simulink model "Admittance"  (R2023b)
settings: Solver=VariableStepAuto  StartTime=0.0  StopTime=1000  RelTol=1e-3
values from neighbouring files (symbols this model uses):
  Bm = 0.8    [Admittance_code.m]
  D = 0.6    [Admittance_code.m]
  J = 2* Jm    (= 1.836e-06)    [Admittance_code.m]
  K = 0.011    [Admittance_code.m]
  Km = K    (= 0.011)    [Admittance_code.m]
  Lw = L    (= 0.00058)    [Admittance_code.m]
  M_inv = 1/J    (= 544662.309368)    [Admittance_code.m]
  Rw = R    (= 1.17)    [Admittance_code.m]
settings Model: Creator=sayeholoumi  LastModifiedBy=sayeholoumi

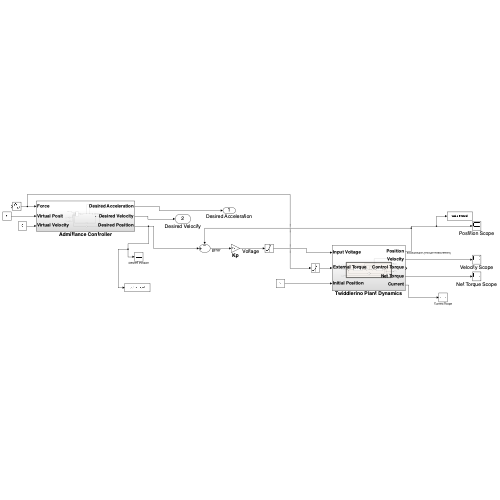
[thumbnail: Simulink's stored preview of the top-level diagram]
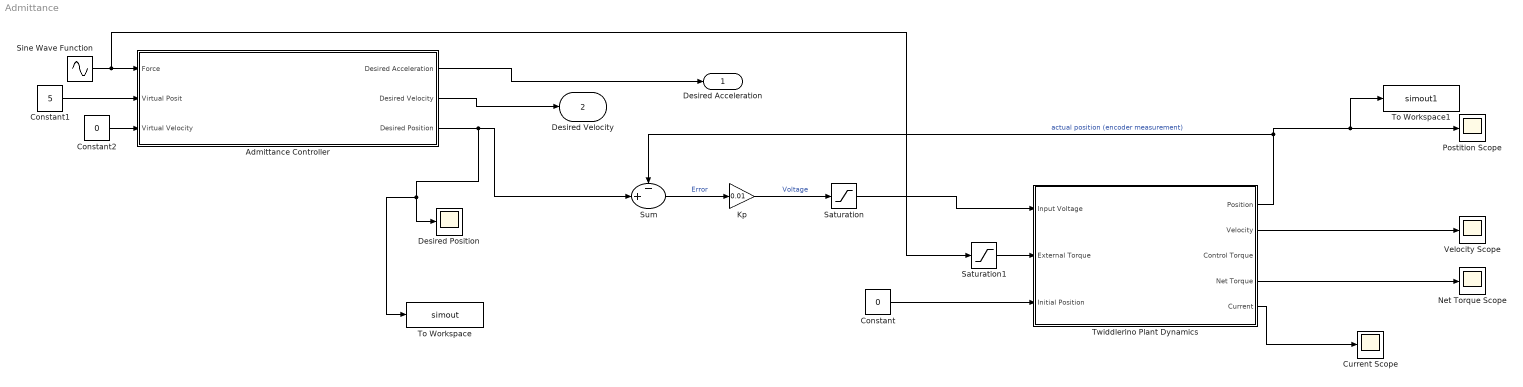
== system Admittance ==
  Admittance Controller : Subsystem
  Constant : Constant  Value=0
  Constant1 : Constant  Value=5
  Constant2 : Constant  Value=0
  Current Scope : Scope
  Desired Position : Scope
  Kp : Gain  Gain=0.01
  Net Torque Scope : Scope
  Postition Scope : Scope
  Saturation : Saturate  UpperLimit=12  LowerLimit=-12
  Saturation1 : Saturate  UpperLimit=12  LowerLimit=-12
  Sine Wave Function : Sin  TimeSource=Use external signal  SampleTime=0
  Sum : Sum  Inputs=-+|
  To Workspace : ToWorkspace  VariableName=simout  SaveFormat=Timeseries  SampleTime=-1
  To Workspace1 : ToWorkspace  VariableName=simout1  SaveFormat=Timeseries  SampleTime=-1
  Twiddlerino Plant Dynamics : Subsystem
  Velocity Scope : Scope
  Desired Acceleration : Outport
  Desired Velocity : Outport  Port=2
  wires:
  Constant/1 -> Twiddlerino Plant Dynamics/3(Initial Position)
  Twiddlerino Plant Dynamics/4(Net Torque) -> Net Torque Scope/1
  Saturation1/1 -> Twiddlerino Plant Dynamics/2(External Torque)
  Saturation/1 -> Twiddlerino Plant Dynamics/1(Input Voltage)
  Sum/1 -> Kp/1  "Error"
  Twiddlerino Plant Dynamics/1(Position) -> Sum/1, To Workspace1/1, Postition Scope/1  "actual position (encoder measurement)"
  Admittance Controller/1(Desired Acceleration) -> Desired Acceleration/1
  Sine Wave Function/1 -> Saturation1/1, Admittance Controller/1(Force)
  Twiddlerino Plant Dynamics/2(Velocity) -> Velocity Scope/1
  Admittance Controller/2(Desired Velocity) -> Desired Velocity/1
  Admittance Controller/3(Desired Position) -> To Workspace/1, Desired Position/1, Sum/2
  Twiddlerino Plant Dynamics/5(Current) -> Current Scope/1
  Kp/1 -> Saturation/1  "Voltage"
  Constant2/1 -> Admittance Controller/3(Virtual Velocity)
  Constant1/1 -> Admittance Controller/2(Virtual Posit)

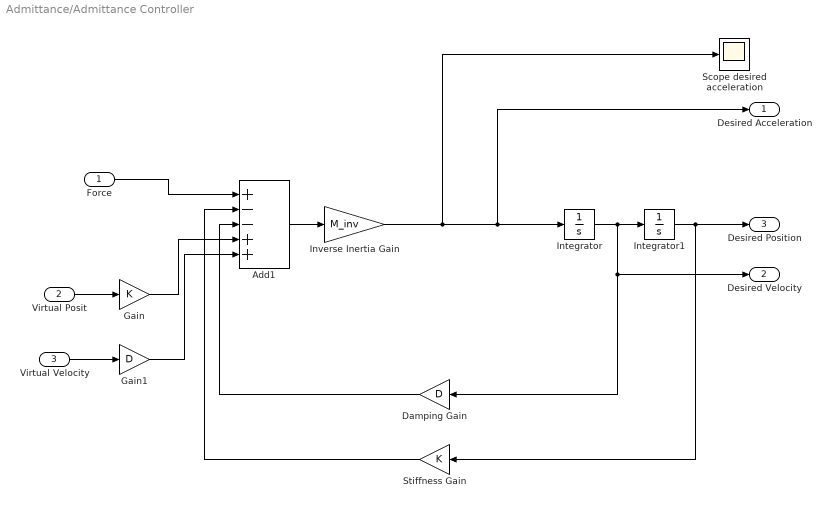
== system Admittance/Admittance Controller ==
  Force : Inport
  Virtual Posit : Inport  Port=2
  Virtual Velocity : Inport  Port=3
  Add1 : Sum  Inputs=+--++
  Damping Gain : Gain  Gain=D
  Gain : Gain  Gain=K
  Gain1 : Gain  Gain=D
  Integrator : Integrator
  Integrator1 : Integrator
  Inverse Inertia Gain : Gain  Gain=M_inv
  Scope desired acceleration : Scope
  "Stiffness Gain " : Gain  Gain=K
  Desired Acceleration : Outport
  Desired Velocity : Outport  Port=2
  Desired Position : Outport  Port=3
  wires:
  Add1/1 -> Inverse Inertia Gain/1
  Damping Gain/1 -> Add1/3
  Integrator1/1 -> Desired Position/1, "Stiffness Gain "/1
  Force/1 -> Add1/1
  Integrator/1 -> Desired Velocity/1, Damping Gain/1, Integrator1/1
  "Stiffness Gain "/1 -> Add1/2
  Inverse Inertia Gain/1 -> Scope desired acceleration/1, Desired Acceleration/1, Integrator/1
  Virtual Posit/1 -> Gain/1
  Virtual Velocity/1 -> Gain1/1
  Gain/1 -> Add1/4
  Gain1/1 -> Add1/5

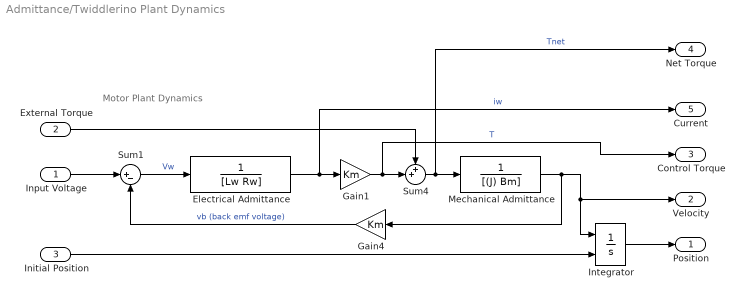
== system Admittance/Twiddlerino Plant Dynamics ==
  note: Motor Plant Dynamics
  Input Voltage : Inport
  External Torque : Inport  Port=2
  Initial Position : Inport  Port=3
  Electrical Admittance : TransferFcn  Denominator=[Lw Rw]
  Gain1 : Gain  Gain=Km
  Gain4 : Gain  Gain=Km
  Integrator : Integrator  InitialConditionSource=external
  Mechanical Admittance : TransferFcn  Denominator=[(J) Bm]
  Sum1 : Sum  Inputs=|+-
  Sum4 : Sum  Inputs=++|
  Position : Outport
  Velocity : Outport  Port=2
  Control Torque : Outport  Port=3
  Net Torque : Outport  Port=4
  Current : Outport  Port=5
  wires:
  Integrator/1 -> Position/1
  Gain1/1 -> Control Torque/1, Sum4/2  "T"
  External Torque/1 -> Sum4/1
  Electrical Admittance/1 -> Current/1, Gain1/1  "iw"
  Initial Position/1 -> Integrator/2
  Mechanical Admittance/1 -> Gain4/1, Integrator/1, Velocity/1
  Sum4/1 -> Net Torque/1, Mechanical Admittance/1  "Tnet"
  Gain4/1 -> Sum1/2  "vb (back emf voltage)"
  Input Voltage/1 -> Sum1/1
  Sum1/1 -> Electrical Admittance/1  "Vw"
